simulink model "Reg_Modal"  (R2017b)
settings: Solver=VariableStepAuto  StartTime=0.0  StopTime=10.0  RelTol=1e-3
values from neighbouring files (symbols this model uses):
  C = [0 1 0 0 0]    [Regul_Luenbergh.m]    (also in Regul_Luenbergh2.m; Regul_Modal.m; Regul_Modal2.m; Regul_Optim.m)
  iv = 2.2    [Regul_Luenbergh.m]    (also in Regul_Luenbergh2.m; Regul_Modal.m; Regul_Modal2.m; Regul_Optim.m)
  k = Q'\(a-az)    [Regul_Luenbergh.m]    (also in Regul_Modal.m = Q'\(a-az),; Regul_Modal2.m)
  k1 = -inv(C/Az*B)    [Regul_Modal.m]    (also in Regul_Modal2.m)
  k1d = -inv(Cd/Az*Bd)    [Regul_Modal2.m]
  kd = Q'\(a-az)    [Regul_Luenbergh2.m]    (also in Regul_Modal2.m)
  Tcn = 0.15    [Regul_Luenbergh.m]    (also in Regul_Luenbergh2.m; Regul_Modal.m; Regul_Modal2.m; Regul_Optim.m)
undefined symbols (not defined in the file or in its folder): Ad, Bd, Cd
settings Model: Creator=ASUS_302  LastModifiedBy=ASUS_302

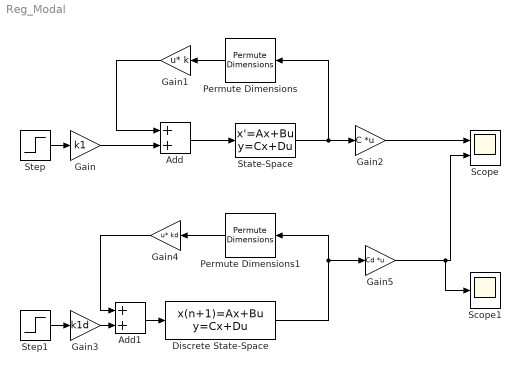
== system Reg_Modal ==
  Add : Sum
  Add1 : Sum
  Discrete State-Space : DiscreteStateSpace  A=Ad  B=Bd  C=eye(5)  D=zeros(5,1)  InitialCondition=[0;0;0;0;0]  SampleTime=0.1
  Gain : Gain  Gain=k1
  Gain1 : Gain  Gain=k  Multiplication=Matrix(u*K)
  Gain2 : Gain  Gain=C  Multiplication=Matrix(K*u)
  Gain3 : Gain  Gain=k1d
  Gain4 : Gain  Gain=kd  Multiplication=Matrix(u*K)
  Gain5 : Gain  Gain=Cd  Multiplication=Matrix(K*u)
  Permute Dimensions : PermuteDimensions
  Permute Dimensions1 : PermuteDimensions
  Scope : Scope  NumInputPorts=2
  Scope1 : Scope
  State-Space : StateSpace  A=|  B=[0; 0; 0; 0; iv/Tcn];  C=eye(5)  D=zeros(5,1)  InitialCondition=[0;0;0;0;0]
      | [c1 c2  0    c3      0;
      |    c4 c5  0    c6     c7;
      |    c8 c9  0    c10    c11;
      |     0  0  1    0       0;
      |     0  0 c12 iv/Tcn -1/Tcn];
  Step : Step  Time=0.01  SampleTime=0
  Step1 : Step  Time=0.01  SampleTime=0
  wires:
  State-Space/1 -> Permute Dimensions/1, Gain2/1
  Gain1/1 -> Add/1
  Gain2/1 -> Scope/1
  Step/1 -> Gain/1
  Gain/1 -> Add/2
  Add/1 -> State-Space/1
  Permute Dimensions/1 -> Gain1/1
  Permute Dimensions1/1 -> Gain4/1
  Discrete State-Space/1 -> Gain5/1, Permute Dimensions1/1
  Gain5/1 -> Scope1/1, Scope/2
  Add1/1 -> Discrete State-Space/1
  Gain4/1 -> Add1/1
  Step1/1 -> Gain3/1
  Gain3/1 -> Add1/2
